simulink model "MotorSysBKP"  (R2019a)
settings: Solver=VariableStepAuto  StartTime=0.0  StopTime=10.0  RelTol=1e-3
undefined symbols (not defined in the file or in its folder): DiscIntNeverNeededParam
libraries: fuzblock x2, simulink x1
settings Model: Creator=936305695  LastModifiedBy=936305695
settings SolverCC: AlgebraicLoopSolver=LineSearch

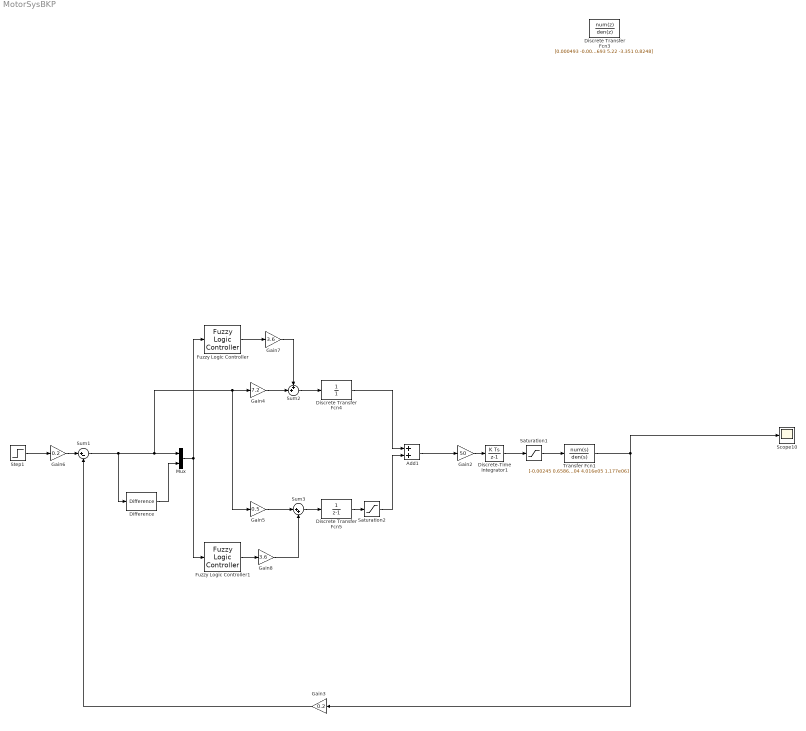
== system MotorSysBKP ==
  Add1 : Sum
  Difference : simulink/Discrete/Difference  ICPrevInput=0.0  OutMin=[]  OutMax=[]  OutDataType=fixdt(1, 16)  OutScaling=2^-10  DoSatur=off
  Discrete Transfer Fcn3 : DiscreteTransferFcn  Numerator=[0.000493 -0.0006711 2.422e-05 0.0001617]  Denominator=[1 -3.693 5.22 -3.351 0.8248]  SampleTime=0.002
  Discrete Transfer Fcn4 : DiscreteTransferFcn  Denominator=[1]  SampleTime=0.002
  Discrete Transfer Fcn5 : DiscreteTransferFcn  Denominator=[1 -1]  SampleTime=0.002
  Discrete-Time Integrator1 : DiscreteIntegrator  SampleTime=0.002  ICPrevOutput=DiscIntNeverNeededParam  ICPrevScaledInput=DiscIntNeverNeededParam
  Fuzzy Logic Controller : fuzblock/Fuzzy Logic  Controller  FIS=mFuzzyKp  OutputSampleNumber=101  DataType=double  FuzzifiedInputs=off  RuleFiringStrengths=off  RuleOutputs=off  AggregatedOutputs=off  SimulateUsing=Interpreted execution  OutOfRangeInputValueMessage=warning  NoRuleFiredMessage=warning  EmptyOutputFuzzySetMessage=warning
  Fuzzy Logic Controller1 : fuzblock/Fuzzy Logic  Controller  FIS=mFuzzyKi  OutputSampleNumber=101  DataType=double  FuzzifiedInputs=off  RuleFiringStrengths=off  RuleOutputs=off  AggregatedOutputs=off  SimulateUsing=Interpreted execution  OutOfRangeInputValueMessage=warning  NoRuleFiredMessage=warning  EmptyOutputFuzzySetMessage=warning
  Gain2 : Gain  Gain=50
  Gain3 : Gain  Gain=0.2
  Gain4 : Gain  Gain=7.2
  Gain5 : Gain  Gain=0.5
  Gain6 : Gain  Gain=0.2
  Gain7 : Gain  Gain=3.6
  Gain8 : Gain  Gain=3.6
  Mux : Mux  Inputs=2
  Saturation1 : Saturate  UpperLimit=5000.0  LowerLimit=-5000.0
  Saturation2 : Saturate  UpperLimit=5.0  LowerLimit=-5.0
  Scope10 : Scope
  Step1 : Step  Time=0  After=150.0  SampleTime=0.002
  Sum1 : Sum  Inputs=|+-
  Sum2 : Sum  Inputs=++|
  Sum3 : Sum  Inputs=|++
  Transfer Fcn1 : TransferFcn  Numerator=[-0.00245 0.6586 77.32 1.65e04 5.995e04]  Denominator=[1 63.17 2.603e04 4.016e05 1.177e06]
  wires:
  Saturation2/1 -> Add1/2
  Discrete Transfer Fcn5/1 -> Saturation2/1
  Add1/1 -> Gain2/1
  Discrete Transfer Fcn4/1 -> Add1/1
  Transfer Fcn1/1 -> Scope10/1, Gain3/1
  Saturation1/1 -> Transfer Fcn1/1
  Discrete-Time Integrator1/1 -> Saturation1/1
  Step1/1 -> Gain6/1
  Gain2/1 -> Discrete-Time Integrator1/1
  Gain3/1 -> Sum1/2
  Sum1/1 -> Difference/1, Gain5/1, Gain4/1, Mux/1
  Gain6/1 -> Sum1/1
  Gain4/1 -> Sum2/2
  Sum2/1 -> Discrete Transfer Fcn4/1
  Gain5/1 -> Sum3/1
  Sum3/1 -> Discrete Transfer Fcn5/1
  Mux/1 -> Fuzzy Logic Controller1/1, Fuzzy Logic Controller/1
  Difference/1 -> Mux/2
  Fuzzy Logic Controller/1 -> Gain7/1
  Gain7/1 -> Sum2/1
  Fuzzy Logic Controller1/1 -> Gain8/1
  Gain8/1 -> Sum3/2
